simulink model "reverse_test2"  (R2023a)
settings: Solver=VariableStepAuto  StartTime=0.0  StopTime=50  RelTol=1e-3
libraries: spsGroundLib x5, spsDCVoltageSourceLib x3, spsIdealSwitchLib x3, spsBreakerLib x3, spsParallelRLCBranchLib x3, spsSeriesRLCBranchLib x2, spsStairGeneratorLib x2, spsDCMachineLib x1, spsVoltageMeasurementLib x1, sps_lib x1
settings Model: Creator=ASUS  LastModifiedBy=ASUS
settings SolverCC: AlgebraicLoopSolver=TrustRegion
settings DebuggingCC: UnconnectedInputMsg=warning  UnconnectedOutputMsg=warning  UnconnectedLineMsg=warning  ArithmeticOperatorsInVariantConditions=warning
settings ModelReferenceCC: EnableRefExpFcnMdlSchedulingChecks=on
settings SFSimCC: CustomCodeUndefinedFunction=UseInterfaceOnly
settings CodeAppCC: StateflowObjectComments=on
settings SimscapeCC: SimscapeNormalizeSystem=off

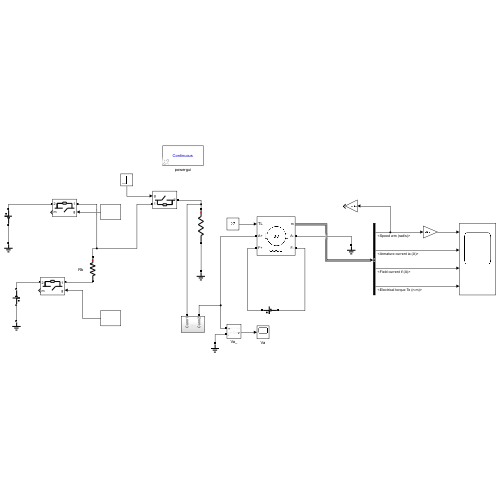
[thumbnail: Simulink's stored preview of the top-level diagram]
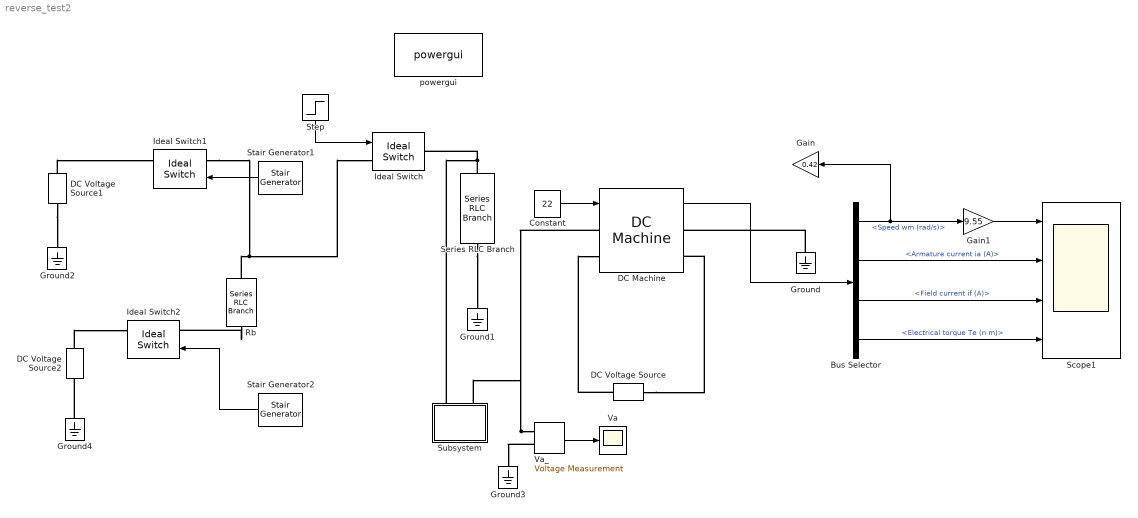
== system reverse_test2 ==
  Bus Selector : BusSelector  OutputSignals=Speed wm (rad/s),Armature current ia (A),Field current if (A),Electrical torque Te (n m)
  Constant : Constant  Value=22
  DC Machine : spsDCMachineLib/DC Machine  PresetModel=No  MechanicalLoad=Torque TL  FieldType=Wound  ShowDetailedParameters=on  MeasurementBus=off  RLa="[ 0.6  0.012]"  RLf="[ 240  120]"  Laf=1.8  MachineConstant=Torque constant (N.m/A)  Ke=1.8  Kt=1.8  J=0.75  Bm=0  Tf=0  w0=1  Ifinit=0.916666666666667  TsPowergui=0  TsBlock=-1
  DC Voltage Source : spsDCVoltageSourceLib/DC Voltage Source  Amplitude=220  Measurements=None
  DC Voltage Source1 : spsDCVoltageSourceLib/DC Voltage Source  Amplitude=220  Measurements=None
  DC Voltage Source2 : spsDCVoltageSourceLib/DC Voltage Source  Amplitude=200  Measurements=None
  Gain : Gain  Gain=0.42
  Gain1 : Gain  Gain=9.55
  Ground{,1..4} (5 alike) : spsGroundLib/Ground  LConnTagsString=a
  Ideal Switch : spsIdealSwitchLib/Ideal Switch  Ron=0.001  Lon=0  IC=0  Rs=1e5  Cs=inf  Measurements=off
  Ideal Switch1 : spsIdealSwitchLib/Ideal Switch  Ron=0  Lon=0  IC=0  Rs=1e5  Cs=inf  Measurements=on
  Ideal Switch2 : spsIdealSwitchLib/Ideal Switch  Ron=0  Lon=0  IC=1  Rs=1e5  Cs=inf  Measurements=on
  Rb : spsSeriesRLCBranchLib/Series RLC Branch  LConnTagsString=__new0  RConnTagsString=__new0  BranchType=R  Resistance=4  Inductance=1e-3  SetiL0=off  InitialCurrent=0  Capacitance=1e-6  Setx0=off  InitialVoltage=0  Measurements=None
  Scope1 : Scope  NumInputPorts=4
  Series RLC Branch : spsSeriesRLCBranchLib/Series RLC Branch  LConnTagsString=__new0  RConnTagsString=__new0  BranchType=R  Resistance=10000  Inductance=1e-3  SetiL0=off  InitialCurrent=0  Capacitance=1e-6  Setx0=off  InitialVoltage=0  Measurements=None
  Stair Generator1 : spsStairGeneratorLib/Stair Generator  t=[0,9]  e=[1,0]  Ts=0
  Stair Generator2 : spsStairGeneratorLib/Stair Generator  t=[9]  e=[1]  Ts=0
  Step : Step  SampleTime=0
  Subsystem : Subsystem
  Va : Scope
  Va_ : spsVoltageMeasurementLib/Voltage Measurement  PhasorSimulation=off  OutputType=Complex  PSBequivalent=0
  powergui : sps_lib/powergui  Priority=1  SimulationMode=Continuous  SampleTime=50e-6  frequency=60  Iterations=50  frequencyindice=0  Pbase=100e6  ErrMax=1e-4  UnitsV=kV  UnitsW=MW  buscounter=0  FunctionMessages=off  echomessages=off  EnableUseOfTLC=off  CurrentSourceSwitches=off  DisableSnubberDevices=off  DisableRonSwitches=off  DisableVfSwitches=off  DisplayEquations=off  AutomaticDiscreteSolvers=off  SolverType=Tustin/Backward Euler (TBE)  Interpol=off  ExternalGateDelay=off  methode=off  Ts=100  x0status=blocks  SPID=on  SwTol=0  HookPort=off  NonlinearTolerance=1e-4  nMaxIteration=100  ContinueOnMaxIteration=off  RestoreLinks=warning  ResistiveCurrentMeasurement=off  Frange=[0:2:500]  Ylog=off  Xlog=on  ShowGrid=off  save=off  variable=ZData  structure=0  ZoomFFT=off  StartTime=0.0  cycles=1  DisplayStyle=1  fundamental=60  FreqAxis=off  MaxFrequency=1000  frequencyindicesteady=1  RmsSteady=1  display=off
  wires:
  Bus Selector/2 -> Scope1/2  "<Armature current ia (A)>"
  Bus Selector/4 -> Scope1/4  "<Electrical torque Te (n m)>"
  Gain1/1 -> Scope1/1
  Bus Selector/3 -> Scope1/3  "<Field current if (A)>"
  Bus Selector/1 -> Gain/1, Gain1/1  "<Speed wm (rad/s)>"
  DC Machine/1 -> Bus Selector/1
  Va_/1 -> Va/1
  Stair Generator2/1 -> Ideal Switch2/1
  Stair Generator1/1 -> Ideal Switch1/1
  Step/1 -> Ideal Switch/1
  Constant/1 -> DC Machine/1
  connections:
  Va_/LConn1 -- DC Machine/LConn1 -- Subsystem/LConn2
  Ideal Switch1/LConn1 -- Rb/LConn1 -- Ideal Switch/LConn1
  Series RLC Branch/LConn1 -- Subsystem/LConn1 -- Ideal Switch/RConn1
  DC Voltage Source/RConn1 -- DC Machine/LConn2
  DC Voltage Source1/RConn1 -- Ideal Switch1/RConn1
  DC Voltage Source/LConn1 -- DC Machine/RConn2
  Series RLC Branch/RConn1 -- Ground1/LConn1
  Va_/LConn2 -- Ground3/LConn1
  DC Voltage Source1/LConn1 -- Ground2/LConn1
  Ground4/LConn1 -- DC Voltage Source2/RConn1
  DC Voltage Source2/LConn1 -- Ideal Switch2/RConn1
  Rb/RConn1 -- Ideal Switch2/LConn1
  Ground/LConn1 -- DC Machine/RConn1

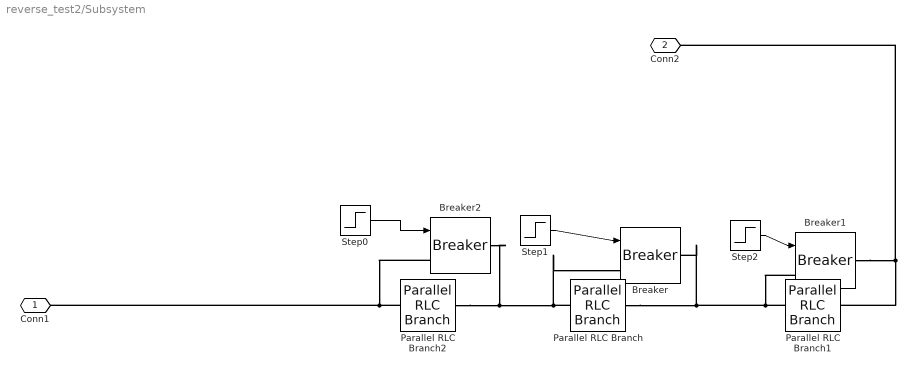
== system reverse_test2/Subsystem ==
  Breaker : spsBreakerLib/Breaker  InitialState=0  SwitchingTimes="[1/60  5/60]"  External=on  BreakerResistance=0.01  SnubberResistance=1e6  SnubberCapacitance=inf  Measurements=None  MoreParameters=on  NoBreakLoop=off
  Breaker1 : spsBreakerLib/Breaker  InitialState=0  SwitchingTimes="[1/60  5/60]"  External=on  BreakerResistance=0.01  SnubberResistance=1e6  SnubberCapacitance=inf  Measurements=None  MoreParameters=on  NoBreakLoop=off
  Breaker2 : spsBreakerLib/Breaker  InitialState=0  SwitchingTimes="[1/60  5/60]"  External=on  BreakerResistance=0.01  SnubberResistance=1e6  SnubberCapacitance=inf  Measurements=None  MoreParameters=on  NoBreakLoop=off
  Parallel RLC Branch : spsParallelRLCBranchLib/Parallel RLC Branch  LConnTagsString=a  RConnTagsString=__new0  BranchType=R  Resistance=0.81  Inductance=1e-3  SetiL0=off  InitialCurrent=0  Capacitance=1e-6  Setx0=off  InitialVoltage=0  Measurements=None
  Parallel RLC Branch1 : spsParallelRLCBranchLib/Parallel RLC Branch  LConnTagsString=a  RConnTagsString=__new0  BranchType=R  Resistance=0.36  Inductance=1e-3  SetiL0=off  InitialCurrent=0  Capacitance=1e-6  Setx0=off  InitialVoltage=0  Measurements=None
  Parallel RLC Branch2 : spsParallelRLCBranchLib/Parallel RLC Branch  LConnTagsString=a  RConnTagsString=__new0  BranchType=R  Resistance=2.4  Inductance=1e-3  SetiL0=off  InitialCurrent=0  Capacitance=1e-6  Setx0=off  InitialVoltage=0  Measurements=None
  Step0 : Step  Time=4.214  SampleTime=0
  Step1 : Step  Time=6.088  SampleTime=0
  Step2 : Step  Time=6.922  SampleTime=0
  Conn1 : PMIOPort  Side=Left
  Conn2 : PMIOPort  Port=2  Side=Left
  wires:
  Step0/1 -> Breaker2/1
  Step2/1 -> Breaker1/1
  Step1/1 -> Breaker/1
  connections:
  Parallel RLC Branch1/LConn1 -- Breaker1/LConn1 -- Parallel RLC Branch/RConn1 -- Breaker/RConn1
  Breaker1/RConn1 -- Conn2/RConn1 -- Parallel RLC Branch1/RConn1
  Parallel RLC Branch2/LConn1 -- Conn1/RConn1 -- Breaker2/LConn1
  Parallel RLC Branch2/RConn1 -- Breaker2/RConn1 -- Parallel RLC Branch/LConn1 -- Breaker/LConn1
